simulink model "Pneumatic_pressure_systems_2015"  (R2015b)
settings: Solver=ode45  SolverMode=SingleTasking  StartTime=0.0  StopTime=4  MaxStep=1e-3  RelTol=1e-3
InitFcn:
  | % 预分配步长数组
  | stepSizes = zeros(1, 10000); % 根据需要调整大小
  | assignin('base', 'stepSizes', stepSizes);
StopFcn:
  | % 将数据存储到工作区
  | stepSizes = evalin('base', 'stepSizes');
  | assignin('base', 'timeStepSizes', stepSizes(stepSizes ~= 0));
undefined symbols (not defined in the file): x, y, z
libraries: fuzblock x1
settings Model: Creator=Administrator  LastModifiedBy=Administrator
settings SolverCC: MaxConsecutiveMinStep=2  ZeroCrossAlgorithm=Adaptive
settings DataIOCC: LimitDataPoints=off  ReturnWorkspaceOutputs=on
settings DebuggingCC: MaskedZcDiagnostic=none  IgnoredZcDiagnostic=none  UnconnectedInputMsg=none  UnconnectedOutputMsg=none  UnconnectedLineMsg=none  AllowSymbolicDim=on  SFUnexpectedBacktrackingDiag=error  SFNoUnconditionalDefaultTransitionDiag=error
settings ModelReferenceCC: EnableRefExpFcnMdlSchedulingChecks=off  PropagateSignalLabelsOutOfModel=on
settings SFSimCC: SimUseLocalCustomCode=on
settings RTWCC: RTWUseLocalCustomCode=on
settings GRTTargetCC: TargetLangStandard=C99 (ISO)
settings ConfigComp: CovMetricSettings=dwe  CovSaveCumulativeToWorkspaceVar=off  CovSaveSingleToWorkspaceVar=off  CovModelRefEnable=Off  CovExternalEMLEnable=on
settings ConfigurationSet: Description=Simscape Multibody

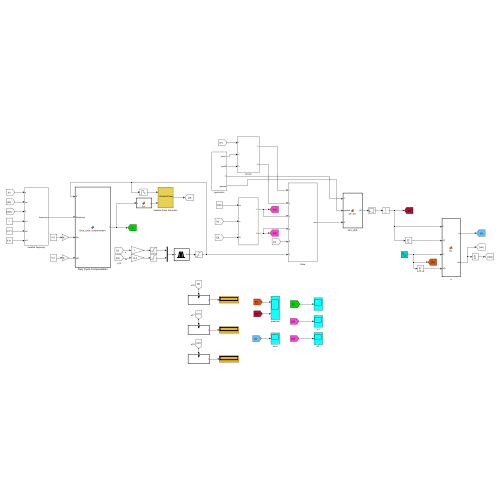
[thumbnail: Simulink's stored preview of the top-level diagram]
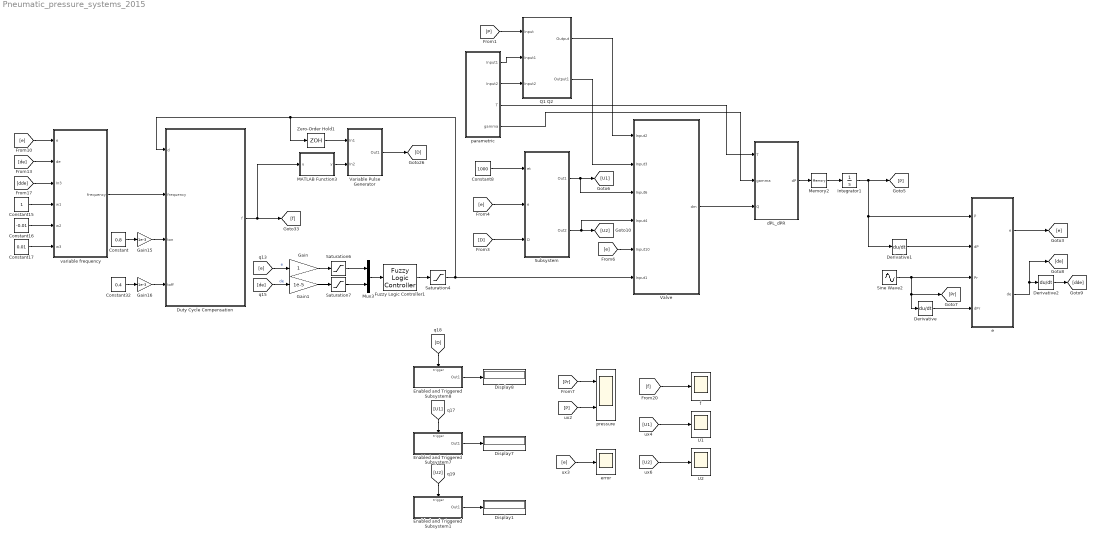
== system Pneumatic_pressure_systems_2015 ==
  Constant : Constant  Value=0.8
  Constant15 : Constant
  Constant16 : Constant  Value=-0.01
  Constant17 : Constant  Value=0.01
  Constant32 : Constant  Value=0.4
  Constant8 : Constant  Value=1000
  Derivative : Derivative
  Derivative1 : Derivative
  Derivative2 : Derivative
  Display1 : Display
  Display7 : Display
  Display8 : Display
  Duty Cycle Compensation : MATLAB Function  TreatAsAtomicUnit=on
  Enabled and Triggered Subsystem1 : Subsystem  TreatAsAtomicUnit=on
  Enabled and Triggered Subsystem7 : Subsystem  TreatAsAtomicUnit=on
  Enabled and Triggered Subsystem8 : Subsystem  TreatAsAtomicUnit=on
  Fuzzy Logic Controller1 : fuzblock/Fuzzy Logic  Controller  FIS="\"fuzzy_pressure.fis\""
  Gain : Gain
  Gain1 : Gain  Gain=1e-5
  Gain15 : Gain  Gain=1e-3
  Gain16 : Gain  Gain=1e-3
  Integrator1 : Integrator  InitialCondition=1.01325e5
  MATLAB Function3 : MATLAB Function  TreatAsAtomicUnit=on
  Memory2 : Memory  X0=10
  Mux3 : Mux  Inputs=2
  Q1 Q2 : Subsystem
  Saturation4 : Saturate  UpperLimit=0.98  LowerLimit=0.1
  Saturation6 : Saturate  UpperLimit=4  LowerLimit=-4
  Saturation7 : Saturate  UpperLimit=35  LowerLimit=-35
  Sine Wave2 : Sin  Amplitude=2.98675e5  Bias=4e5  Frequency=2*pi*0.5  SampleTime=0
  Subsystem : Subsystem
  U1 : Scope
  "U2 " : Scope
  Valve : Subsystem
  Variable Pulse Generator : Subsystem  Description=Replaced Block  mask(Replaced Block){}
      mask help: 此模块已被替换为空子系统，因为它使用了在 Simulink R2015b 中不可用的功能。
      mask Display: fprintf('Replaced: %s\n','VariablePulseGenerator')
  Zero-Order Hold1 : ZeroOrderHold  SampleTime=0.01
  dPL_dPR : MATLAB Function  TreatAsAtomicUnit=on
  e : MATLAB Function  TreatAsAtomicUnit=on
  error : Scope
  f : Scope
  parametric : Subsystem
  pressure : Scope  NumInputPorts=2
  variable frequency : Subsystem
  wires:
  dPL_dPR/1(dP) -> Memory2/1
  Valve/1(dm) -> dPL_dPR/3(Q)
  Integrator1/1 -> Derivative1/1, e/1(P), [P]
  Memory2/1 -> Integrator1/1
  [P] -> Q1 Q2/1(Input)
  Derivative/1 -> e/4(dPr)
  Derivative1/1 -> e/2(dP)
  e/2(de) -> [de], Derivative2/1
  MATLAB Function3/1(y) -> Variable Pulse Generator/2(In2)
  Derivative2/1 -> [dde]
  Mux3/1 -> Fuzzy Logic Controller1/1
  [e] -> Gain/1  "e"
  [de] -> Gain1/1  "de"
  Fuzzy Logic Controller1/1 -> Saturation4/1
  Saturation4/1 -> Zero-Order Hold1/1, Duty Cycle Compensation/1(d), Valve/6(Input1)
  Saturation6/1 -> Mux3/1
  Saturation7/1 -> Mux3/2
  Gain/1 -> Saturation6/1
  Gain1/1 -> Saturation7/1
  Constant/1 -> Gain15/1
  Constant32/1 -> Gain16/1
  Gain15/1 -> Duty Cycle Compensation/3(ton)
  Gain16/1 -> Duty Cycle Compensation/4(toff)
  Variable Pulse Generator/1(Out1) -> [D]
  Enabled and Triggered Subsystem7/1(Out1) -> Display7/1
  Enabled and Triggered Subsystem8/1(Out1) -> Display8/1
  [U2] -> Enabled and Triggered Subsystem1/Trigger
  Enabled and Triggered Subsystem1/1(Out1) -> Display1/1
  [U1] -> Enabled and Triggered Subsystem7/Trigger
  [D] -> Enabled and Triggered Subsystem8/Trigger
  [Pr] -> pressure/1
  [e] -> error/1
  [f] -> f/1
  Zero-Order Hold1/1 -> Variable Pulse Generator/1(In1)
  [U1] -> U1/1
  [P] -> pressure/2
  e/1(e) -> [e]
  Duty Cycle Compensation/1(f) -> MATLAB Function3/1(u), [f]
  Q1 Q2/1(Output) -> Valve/1(Input2)
  Q1 Q2/2(Output1) -> Valve/2(Input3)
  [e] -> variable frequency/1(e)
  [de] -> variable frequency/2(de)
  [dde] -> variable frequency/3(In3)
  Constant15/1 -> variable frequency/4(w1)
  Constant16/1 -> variable frequency/5(w2)
  Constant17/1 -> variable frequency/6(w3)
  variable frequency/1(frequency) -> Duty Cycle Compensation/2(frequency)
  Constant8/1 -> Subsystem/1(et)
  [D] -> Subsystem/3(D)
  [e] -> Subsystem/2(e)
  [e] -> Valve/5(Input10)
  Subsystem/1(Out1) -> Valve/3(Input6), [U1]
  Subsystem/2(Out2) -> Valve/4(Input4), [U2]
  Sine Wave2/1 -> Derivative/1, [Pr], e/3(Pr)
  [U2] -> "U2 "/1
  parametric/1(Input1) -> Q1 Q2/2(Input1)
  parametric/2(Input2) -> Q1 Q2/3(Input2)
  parametric/3(T) -> dPL_dPR/1(T)
  parametric/4(gamma) -> dPL_dPR/2(gamma)

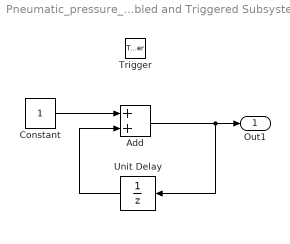
== system Pneumatic_pressure_systems_2015/Enabled and Triggered Subsystem1 ==
  Trigger : TriggerPort
  Add : Sum
  Constant : Constant
  Unit Delay : UnitDelay  SampleTime=-1  HasFrameUpgradeWarning=on
  Out1 : Outport
  wires:
  Unit Delay/1 -> Add/2
  Add/1 -> Out1/1, Unit Delay/1
  Constant/1 -> Add/1

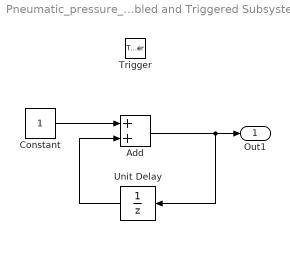
== system Pneumatic_pressure_systems_2015/Enabled and Triggered Subsystem7 ==
  Trigger : TriggerPort
  Add : Sum
  Constant : Constant
  Unit Delay : UnitDelay  SampleTime=-1  HasFrameUpgradeWarning=on
  Out1 : Outport
  wires:
  Constant/1 -> Add/1
  Add/1 -> Unit Delay/1, Out1/1
  Unit Delay/1 -> Add/2

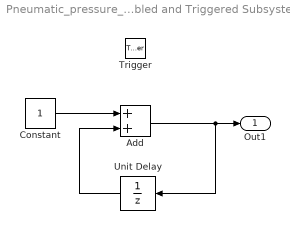
== system Pneumatic_pressure_systems_2015/Enabled and Triggered Subsystem8 ==
  Trigger : TriggerPort
  Add : Sum
  Constant : Constant
  Unit Delay : UnitDelay  SampleTime=-1  HasFrameUpgradeWarning=on
  Out1 : Outport
  wires:
  Unit Delay/1 -> Add/2
  Add/1 -> Out1/1, Unit Delay/1
  Constant/1 -> Add/1

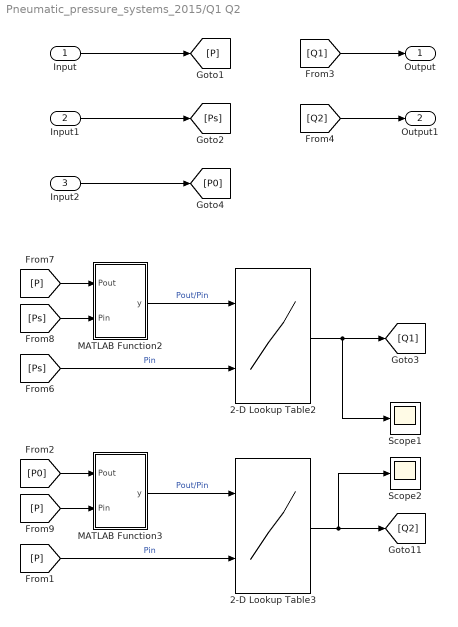
== system Pneumatic_pressure_systems_2015/Q1 Q2 ==
  Input : Inport
  Input1 : Inport  Port=2
  Input2 : Inport  Port=3
  2-D Lookup Table2 : Lookup_n-D  BreakpointsForDimension1=y  BreakpointsForDimension2=x  Table=z  InterpMethod=Cubic spline  ExtrapMethod=Cubic spline  InternalRulePriority=Speed  RndMeth=Simplest  InputSameDT=on
  2-D Lookup Table3 : Lookup_n-D  BreakpointsForDimension1=y  BreakpointsForDimension2=x  Table=z  InterpMethod=Cubic spline  ExtrapMethod=Cubic spline  InternalRulePriority=Speed  RndMeth=Simplest  InputSameDT=on
  MATLAB Function2 : MATLAB Function  TreatAsAtomicUnit=on
  MATLAB Function3 : MATLAB Function  TreatAsAtomicUnit=on
  Scope1 : Scope
  Scope2 : Scope
  Output : Outport
  Output1 : Outport  Port=2
  wires:
  2-D Lookup Table3/1 -> Scope2/1, [Q2]
  [P] -> MATLAB Function2/1(Pout)
  [P0] -> MATLAB Function3/1(Pout)
  MATLAB Function2/1(y) -> 2-D Lookup Table2/1  "Pout/Pin"
  [Ps] -> 2-D Lookup Table2/2  "Pin"
  MATLAB Function3/1(y) -> 2-D Lookup Table3/1  "Pout/Pin"
  2-D Lookup Table2/1 -> Scope1/1, [Q1]
  [P] -> 2-D Lookup Table3/2  "Pin"
  [P] -> MATLAB Function3/2(Pin)
  [Ps] -> MATLAB Function2/2(Pin)
  Input/1 -> [P]
  Input1/1 -> [Ps]
  Input2/1 -> [P0]
  [Q1] -> Output/1
  [Q2] -> Output1/1

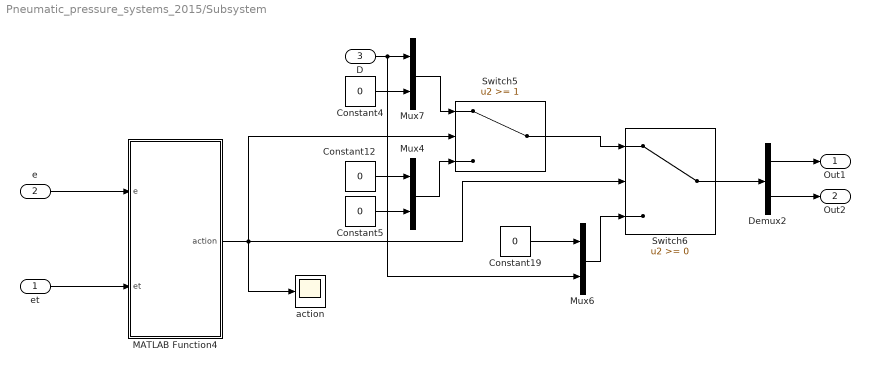
== system Pneumatic_pressure_systems_2015/Subsystem ==
  et : Inport
  e : Inport  Port=2
  D : Inport  Port=3
  Constant{4..5,12,19} (4 alike) : Constant  Value=0
  Demux2 : Demux  Outputs=2
  MATLAB Function4 : MATLAB Function  TreatAsAtomicUnit=on  SystemSampleTime=0.001
  Mux4 : Mux  Inputs=2
  Mux6 : Mux  Inputs=2
  Mux7 : Mux  Inputs=2
  Switch5 : Switch  Threshold=1
  Switch6 : Switch
  action : Scope
  Out1 : Outport
  Out2 : Outport  Port=2
  wires:
  Switch5/1 -> Switch6/1
  MATLAB Function4/1(action) -> Switch5/2, Switch6/2, action/1
  Constant4/1 -> Mux7/2
  Mux4/1 -> Switch5/3
  Constant5/1 -> Mux4/2
  D/1 -> Mux6/2, Mux7/1
  Switch6/1 -> Demux2/1
  Mux7/1 -> Switch5/1
  Mux6/1 -> Switch6/3
  Constant12/1 -> Mux4/1
  Constant19/1 -> Mux6/1
  et/1 -> MATLAB Function4/2(et)
  Demux2/1 -> Out1/1
  Demux2/2 -> Out2/1
  e/1 -> MATLAB Function4/1(e)

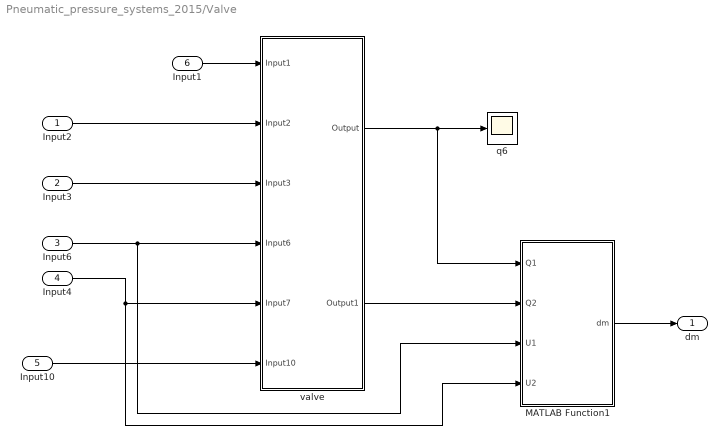
== system Pneumatic_pressure_systems_2015/Valve ==
  Input2 : Inport
  Input3 : Inport  Port=2
  Input6 : Inport  Port=3
  Input4 : Inport  Port=4
  Input10 : Inport  Port=5
  Input1 : Inport  Port=6
  MATLAB Function1 : MATLAB Function  TreatAsAtomicUnit=on
  q6 : Scope
  valve : Subsystem
  dm : Outport
  wires:
  Input2/1 -> valve/2(Input2)
  Input6/1 -> MATLAB Function1/3(U1), valve/4(Input6)
  Input4/1 -> valve/5(Input7), MATLAB Function1/4(U2)
  Input1/1 -> valve/1(Input1)
  valve/1(Output) -> MATLAB Function1/1(Q1), q6/1
  MATLAB Function1/1(dm) -> dm/1
  valve/2(Output1) -> MATLAB Function1/2(Q2)
  Input10/1 -> valve/6(Input10)
  Input3/1 -> valve/3(Input3)

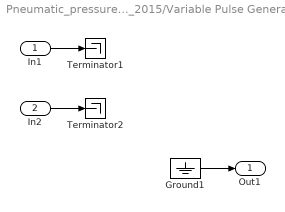
== system Pneumatic_pressure_systems_2015/Variable Pulse Generator ==
  In1 : Inport
  In2 : Inport  Port=2
  Ground1 : Ground
  Terminator1 : Terminator
  Terminator2 : Terminator
  Out1 : Outport
  wires:
  Ground1/1 -> Out1/1
  In2/1 -> Terminator2/1
  In1/1 -> Terminator1/1

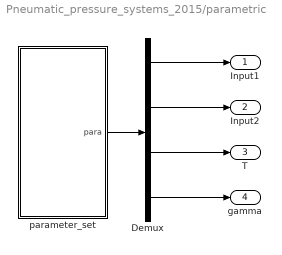
== system Pneumatic_pressure_systems_2015/parametric ==
  Demux : Demux
  parameter_set : MATLAB Function  TreatAsAtomicUnit=on
  Input1 : Outport
  Input2 : Outport  Port=2
  T : Outport  Port=3
  gamma : Outport  Port=4
  wires:
  Demux/2 -> Input2/1
  parameter_set/1(para) -> Demux/1
  Demux/4 -> gamma/1
  Demux/3 -> T/1
  Demux/1 -> Input1/1

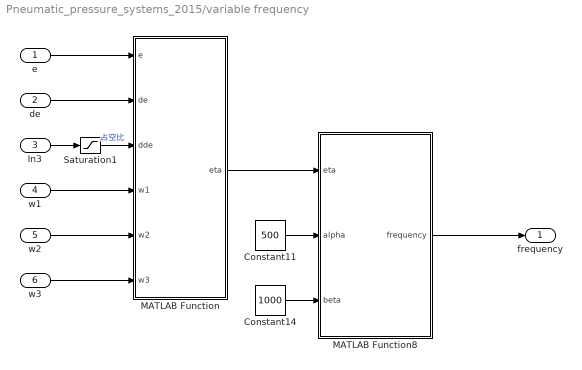
== system Pneumatic_pressure_systems_2015/variable frequency ==
  e : Inport
  de : Inport  Port=2
  In3 : Inport  Port=3
  w1 : Inport  Port=4
  w2 : Inport  Port=5
  w3 : Inport  Port=6
  Constant11 : Constant  Value=500
  Constant14 : Constant  Value=1000
  MATLAB Function : MATLAB Function  TreatAsAtomicUnit=on
  MATLAB Function8 : MATLAB Function  TreatAsAtomicUnit=on
  Saturation1 : Saturate  UpperLimit=1e6  LowerLimit=0  ZeroCross=off
  frequency : Outport
  wires:
  Constant11/1 -> MATLAB Function8/2(alpha)
  Constant14/1 -> MATLAB Function8/3(beta)
  Saturation1/1 -> MATLAB Function/3(dde)  "占空比"
  MATLAB Function8/1(frequency) -> frequency/1
  In3/1 -> Saturation1/1
  de/1 -> MATLAB Function/2(de)
  w1/1 -> MATLAB Function/4(w1)
  MATLAB Function/1(eta) -> MATLAB Function8/1(eta)
  e/1 -> MATLAB Function/1(e)
  w2/1 -> MATLAB Function/5(w2)
  w3/1 -> MATLAB Function/6(w3)

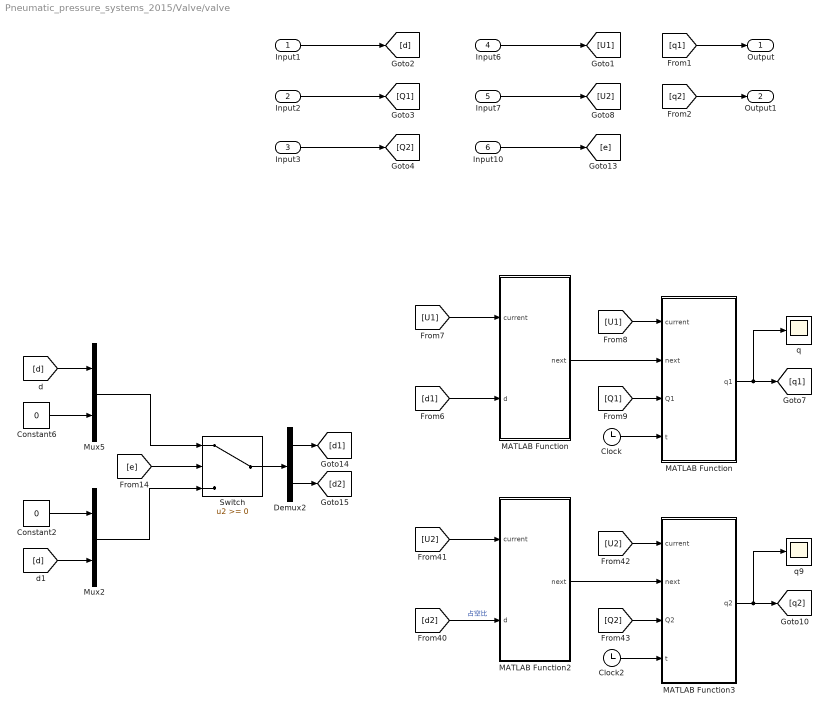
== system Pneumatic_pressure_systems_2015/Valve/valve ==
  Input1 : Inport
  Input2 : Inport  Port=2
  Input3 : Inport  Port=3
  Input6 : Inport  Port=4
  Input7 : Inport  Port=5
  Input10 : Inport  Port=6
  " MATLAB Function" : MATLAB Function  TreatAsAtomicUnit=on
  " MATLAB Function2" : MATLAB Function  TreatAsAtomicUnit=on
  Clock : Clock
  Clock2 : Clock
  Constant2 : Constant  Value=0
  Constant6 : Constant  Value=0
  Demux2 : Demux  Outputs=2
  MATLAB Function : MATLAB Function  TreatAsAtomicUnit=on
  MATLAB Function3 : MATLAB Function  TreatAsAtomicUnit=on
  Mux2 : Mux  Inputs=2
  Mux5 : Mux  Inputs=2
  Switch : Switch
  q : Scope
  q9 : Scope
  Output : Outport
  Output1 : Outport  Port=2
  wires:
  Clock2/1 -> MATLAB Function3/4(t)
  [U1] -> " MATLAB Function"/1(current)
  Clock/1 -> MATLAB Function/4(t)
  [Q1] -> MATLAB Function/3(Q1)
  [d1] -> " MATLAB Function"/2(d)
  MATLAB Function/1(q1) -> q/1, [q1]
  " MATLAB Function"/1(next) -> MATLAB Function/2(next)
  [Q2] -> MATLAB Function3/3(Q2)
  [U1] -> MATLAB Function/1(current)
  MATLAB Function3/1(q2) -> [q2], q9/1
  [U2] -> " MATLAB Function2"/1(current)
  [d2] -> " MATLAB Function2"/2(d)  "占空比"
  " MATLAB Function2"/1(next) -> MATLAB Function3/2(next)
  [U2] -> MATLAB Function3/1(current)
  Input1/1 -> [d]
  Input3/1 -> [Q2]
  Input2/1 -> [Q1]
  [q1] -> Output/1
  [q2] -> Output1/1
  Input7/1 -> [U2]
  Input6/1 -> [U1]
  Input10/1 -> [e]
  Mux2/1 -> Switch/3
  Mux5/1 -> Switch/1
  Constant6/1 -> Mux5/2
  [d] -> Mux2/2
  Demux2/1 -> [d1]
  Switch/1 -> Demux2/1
  Constant2/1 -> Mux2/1
  [e] -> Switch/2
  [d] -> Mux5/1
  Demux2/2 -> [d2]

== matlab function Pneumatic_pressure_systems_2015/Q1 Q2/MATLAB Function3 ==
  data: Pout input; y output; Pin input
function y = fcn(Pout,Pin)

y=Pout/Pin;

== matlab function Pneumatic_pressure_systems_2015/e ==
  data: P input; dP input; e output; Pr input; dPr input; de output
function [e,de]= fcn(P,dP,Pr,dPr)

e = Pr-P;
de=dPr-dP;

== matlab function Pneumatic_pressure_systems_2015/Q1 Q2/MATLAB Function2 ==
  data: Pout input; y output; Pin input
function y = fcn(Pout,Pin)

y=Pout/Pin;

== matlab function Pneumatic_pressure_systems_2015/Valve/MATLAB Function1 ==
  data: dm output; Q1 input; Q2 input; U1 input; U2 input
function dm = flow_calculate(Q1,Q2,U1,U2)

 dm =U1*Q1 -U2*Q2;

== matlab function Pneumatic_pressure_systems_2015/dPL_dPR ==
  data: dP output size=1; T input; gamma input; Q input
function dP  = dP_fun(T,gamma,Q)

R=0.287;
V=1.57e-4;

dP = gamma*R*T*Q/V;

== matlab function Pneumatic_pressure_systems_2015/Subsystem/MATLAB Function4 ==
  data: e input; action output; et input
function action= control_test(e,et)
        

if e>et    
    action = 1;      
else        
       
    if e>=-et && e<=et
         action = 0;    
    else
         if e<-et
               action = -1;  
         else
          action=0;   
        end
    end
end

== matlab function Pneumatic_pressure_systems_2015/variable frequency/MATLAB Function ==
  data: e input; eta output; de input; dde input; w1 input; w2 input; w3 input
function eta = fcn(e,de,dde,w1,w2,w3)   % w1,w2,w3 三个参数 具体大小怎么确定

%w1=1;        %三个参数w1,w2,w3
%w2=0.5;
%w3=1;

eta = w1*e+w2*de+w3*dde;

== matlab function Pneumatic_pressure_systems_2015/parametric/parameter_set ==
  data: para output
function para = parameter_set()  %parameter 变量
global t0_1 t0_2 t0_3 t0_4 flag1 flag2 flag3 flag4;
para = 1:4;  

Ps = 8e5;
P0 = 1.01325e5;
T=  293.15;
gamma =1.4;                



para(1) = Ps;           
para(2) = P0;
para(3) = T;
para(4) = gamma;

== matlab function Pneumatic_pressure_systems_2015/variable frequency/MATLAB Function8 ==
  data: frequency output; eta input; alpha input; beta input
function frequency = fcn(eta,alpha,beta)   %问题：高频、中频、低频 具体大小怎么确定
                                                % alpha，beta 两个参数 具体大小怎么确定

frequency = 500;


%alpha = 0.05;    %alpha，beta 是两个参数
%beta  = 0.1;


if eta >= beta 
    frequency = 100;             %低频
else
    if eta >= alpha && eta < beta
        frequency = 300;         %中频
    else
        if eta >= -alpha &&  eta < alpha
            frequency = 500;     %高频
        else
            if  eta >= -beta &&  eta <-alpha
                frequency = 300; %中频
            else
                 if  eta <-beta
                frequency = 100; %低频
                 else
                 end
            end
        end
    end
end

== matlab function Pneumatic_pressure_systems_2015/MATLAB Function3 ==
  data: u input; y output
function y = fcn(u)

y = 1/u;

== matlab function Pneumatic_pressure_systems_2015/Duty Cycle Compensation ==
  data: f output; d input; frequency input; ton input; toff input
function f = Duty_cycle_compensation(d, frequency,ton,toff)
    
  
    if frequency == 500
        if ton*500 <= d && d <= 1-toff*500
            f = 500;
        elseif ton*300 <= d && d <= 1-toff*300
            f = 300;
        else
            f = 100; 
        end
    elseif frequency == 300
        if ton*300 <= d && d <= 1-toff*300
            f = 300;
        else
            f = 100;
        end
    else 
        f = 100; 
    end
end

== matlab function Pneumatic_pressure_systems_2015/Valve/valve/ MATLAB Function ==
  settings: updateMethod=DISCRETE
  data: current input; next output; d input
function next = getNextPWMLevel(current, d)
 
    
    if current == 0
        if rand <= d
            next = 1;
        else
            next = 0;
        end
    else
        if rand <= (1 - d)
            next = 0;
        else
            next = 1;
        end
    end
end

== matlab function Pneumatic_pressure_systems_2015/Valve/valve/ MATLAB Function2 ==
  settings: updateMethod=DISCRETE
  data: current input; next output; d input
function next = getNextPWMLevel(current, d)
  
    
    if current == 0
        if rand <= d
            next = 1;
        else
            next = 0;
        end
    else
        if rand <= (1 - d)
            next = 0;
        else
            next = 1;
        end
    end
end

== matlab function Pneumatic_pressure_systems_2015/Valve/valve/MATLAB Function ==
  data: current input; q1 output; next input; Q1 input; t input
function q1= lag(current,next,Q1,t)
period=0.55e-3; 
mode = 0;
flag1 = 1;

if (current == 0 && next == 0) || (current == 1 && next == 1)
    mode = 0;
end
if current == 0 && next == 1
    mode =1;
end
if current == 1 && next == 0
    mode =2;
end

switch(mode)
    case 0
        q1   = Q1; 
    case 1        
        if flag1 == 1
            t0_1 = t;
            flag1 = 0;
        end
        t1 = t - t0_1;
        if t1<=period
            q1 = Q1/period*t1;
        else
            q1 = Q1;
            flag1 = 1;
        end
        
    case 2       
        if flag1 == 1
            t0_1 = t;
           flag1 = 0;
        end
        t1 = t - t0_1;
        
        if t1<=period
            q1 = Q1/period*(period - t1);
        else
            q1 = Q1;
            flag1 = 1;
        end
    otherwise
        q1 = Q1;
end

== matlab function Pneumatic_pressure_systems_2015/Valve/valve/MATLAB Function3 ==
  data: current input; q2 output; next input; Q2 input; t input
function q2= lag(current,next,Q2,t)
period=0.55e-3; 

mode = 0;
flag2 = 1;

if (current == 0 && next == 0) || (current == 1 && next == 1)
    mode = 0;
end
if current == 0 && next == 1
    mode =1;
end
if current == 1 && next == 0
    mode =2;
end

switch(mode)
    case 0
        q2   = Q2;  
    case 1        
        if flag2 == 1
            t0_2 = t;
            flag2 = 0;
        end
        t1 = t - t0_2;
        if t1<=period
            q2 = Q2/period*t1;
        else
            q2 = Q2;
            flag2 = 1;
        end
        
    case 2      
        if flag2 == 1
            t0_2 = t;
           flag2 = 0;
        end
        t1 = t - t0_2;
        
        if t1<=period
            q2 = Q2/period*(period - t1);
        else
            q2 = Q2;
            flag2 = 1;
        end
    otherwise
        q2 = Q2;
end
